simulink model "pure_inematic"  (R2020b)
settings: Solver=FixedStepAuto  StartTime=0.0  StopTime=40  FixedStep=0.001  RelTol=1e-3
settings Model: Creator=cyx  LastModifiedBy=cyx
settings DataIOCC: ReturnWorkspaceOutputs=off

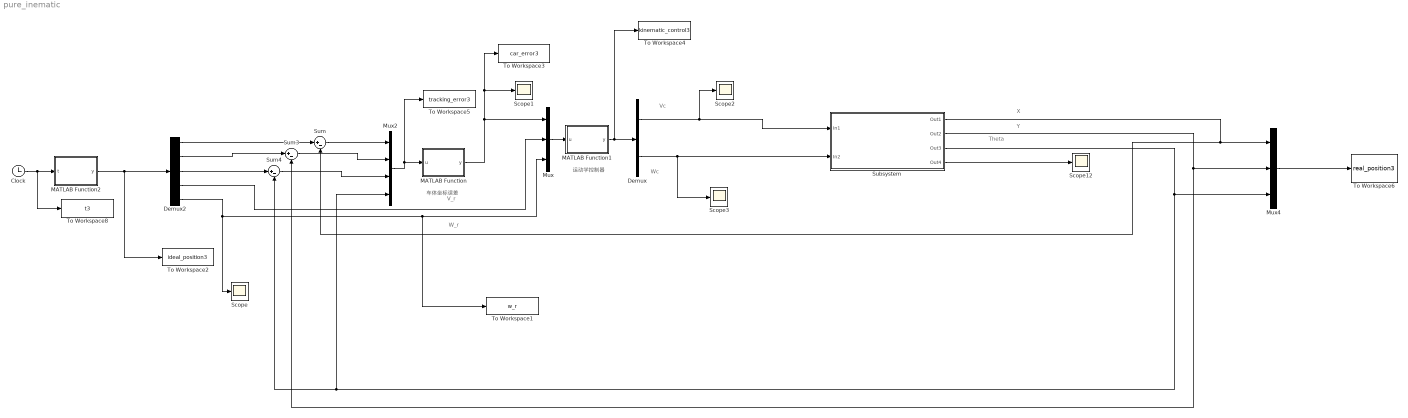
== system pure_inematic ==
  note: 运动学控制器
  note: Theta
  note: Wc
  note: X
  note: V_r
  note: Vc
  note: W_r
  note: 车体坐标误差
  note: Y
  Clock : Clock
  Demux : Demux  Outputs=[1 1]
  Demux2 : Demux  Outputs=5
  MATLAB Function : MATLAB Function  TreatAsAtomicUnit=on
  MATLAB Function1 : MATLAB Function  TreatAsAtomicUnit=on
  MATLAB Function2 : MATLAB Function  TreatAsAtomicUnit=on
  Mux : Mux  Inputs=3
  Mux2 : Mux  Inputs=[1 1 1 1]
  Mux4 : Mux  Inputs=3
  Scope{,1..3,12} (5 alike) : Scope
  Subsystem : Subsystem
  Sum : Sum  Inputs=|+-
  Sum3 : Sum  Inputs=|+-
  Sum4 : Sum  Inputs=|+-
  To Workspace1 : ToWorkspace  VariableName=w_r  SampleTime=-1
  To Workspace2 : ToWorkspace  VariableName=ideal_position3  SampleTime=-1
  To Workspace3 : ToWorkspace  VariableName=car_error3  SampleTime=-1
  To Workspace4 : ToWorkspace  VariableName=kinematic_control3  SampleTime=-1
  To Workspace5 : ToWorkspace  VariableName=tracking_error3  SampleTime=-1
  To Workspace6 : ToWorkspace  VariableName=real_position3  SampleTime=-1
      settings: Save2DSignal=2-D array (concatenate along first dimension)
  To Workspace8 : ToWorkspace  VariableName=t3  SampleTime=-1
  wires:
  Mux4/1 -> To Workspace6/1
  Demux2/3 -> Sum4/1
  Subsystem/1(Out1) -> Mux4/1, Sum/2
  MATLAB Function2/1(y) -> To Workspace2/1, Demux2/1
  Demux2/4 -> Mux/2
  Clock/1 -> To Workspace8/1, MATLAB Function2/1(t)
  Subsystem/3(Out3) -> Mux4/3, Mux2/4, Sum4/2
  Sum/1 -> Mux2/1
  Subsystem/4(Out4) -> Scope12/1
  Sum3/1 -> Mux2/2
  Mux2/1 -> To Workspace5/1, MATLAB Function/1(u)
  Sum4/1 -> Mux2/3
  Demux2/1 -> Sum/1
  Mux/1 -> MATLAB Function1/1(u)
  Demux2/2 -> Sum3/1
  Subsystem/2(Out2) -> Mux4/2, Sum3/2
  MATLAB Function/1(y) -> To Workspace3/1, Scope1/1, Mux/1
  MATLAB Function1/1(y) -> To Workspace4/1, Demux/1
  Demux/1 -> Scope2/1, Subsystem/1(In1)
  Demux/2 -> Scope3/1, Subsystem/2(In2)
  Demux2/5 -> To Workspace1/1, Mux/3, Scope/1

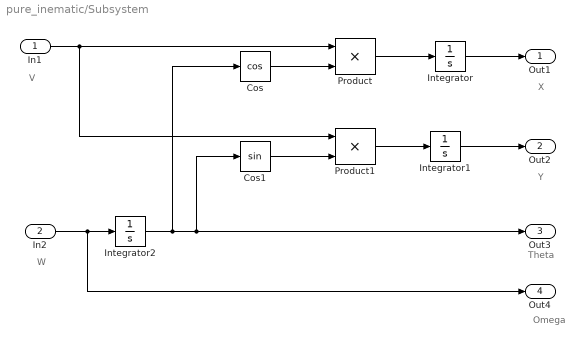
== system pure_inematic/Subsystem ==
  note: W
  note: V
  note: X
  note: Y
  note: Theta
  note: Omega
  In1 : Inport
  In2 : Inport  Port=2
  Cos : Trigonometry  Operator=cos
  Cos1 : Trigonometry
  Integrator : Integrator  InitialCondition=-2
  Integrator1 : Integrator  InitialCondition=-2
  Integrator2 : Integrator
  Product : Product
  Product1 : Product
  Out1 : Outport
  Out2 : Outport  Port=2
  Out3 : Outport  Port=3
  Out4 : Outport  Port=4
  wires:
  In1/1 -> Product1/1, Product/1
  Product/1 -> Integrator/1
  Integrator/1 -> Out1/1
  Cos/1 -> Product/2
  Integrator1/1 -> Out2/1
  In2/1 -> Out4/1, Integrator2/1
  Integrator2/1 -> Cos1/1, Out3/1, Cos/1
  Product1/1 -> Integrator1/1
  Cos1/1 -> Product1/2

== matlab function pure_inematic/MATLAB Function ==
  data: u input; y output
function y = error(u)
%%讲机器人误差坐标进行转换；
%转换矩阵C

C=[cos(u(4))   sin(u(4))    0;
   -sin(u(4)) cos(u(4))    0;
    0            0          1];

%%将世界坐标系下的误差转化至车体坐标下转换后的误差q_e=[e1 e2 e3]
%输入为世界坐标系下的误差x_e,y_e,theta_e对应u(1),u(2) u(3)
e1=C(1,1)*u(1)+C(1,2)*u(2);
e2=C(2,1)*u(1)+C(2,2)*u(2);
e3=C(3,3)*u(3);
y =[e1;e2;e3];

== matlab function pure_inematic/MATLAB Function2 ==
  data: t input; y output
function y = input(t)

S=3;
switch S

   case 1 %圆形轨迹
       w_r=1;
       x_r= 5*cos(w_r*t);
       y_r= 5+5*sin(w_r*t);
       theta_r=w_r*t;
        v_r=5;
               
    case 2 %8轨迹
        x_r=10*sin(t/10);
        y_r=10*sin(t/20);
        dx_r=cos(t/10);
        dy_r=0.5*cos(t/20);
        if atan2(dy_r,dx_r)>0
            theta_r=atan2(dy_r,dx_r);
        else
            theta_r=atan2(dy_r,dx_r)+2*pi;
        end
        v_r=sqrt(dy_r.^2+dx_r.^2);
        w_r=0.5;

    case 3 %rectangle
        x_r=sign(cos(t)).*sqrt(abs(100*cos(t)));
        y_r=sign(sin(t)).*sqrt(abs(100*sin(t)));
        theta_r=atan2(y_r,x_r);
        if 0<t && t<3.146 | 10<t && t<13.146 | 20<t && t<23.146 | 30<t && t<33.146
            v_r=0.8;
            w_r=0.5;
        else
            v_r=1;
            w_r=0;
        end
 
end


y =[x_r; y_r; theta_r; v_r; w_r];

== matlab function pure_inematic/MATLAB Function1 ==
  data: u input; y output
function y = kinematic(u)
ex=u(1);
ey=u(2);
etheta=u(3);
v_r=u(4);
w_r=u(5);
%%机器人反演控制律；控制输入为参考速度v_r,w_r以及三个车体坐标系误差；
%k1=123; k2=1;k3=23;
%v_c=v_r*cos(etheta)+k1*ex;
%w_c=w_r+k2*v_r*ey+k3*v_r*sin(etheta);

%k1=0.01;k2=16;k3=4;k4=16;vr_dot=0;wr_dot=0;
%w_c=k2*ey*v_r*cos(etheta/2)*cos(etheta/4)+w_r+k4*sin(etheta/4);
%v_c=v_r*cos(etheta)-k1*ey/(1+w_c.^2)*(k2*((-w_c*ex+v_r*sin(etheta)*v_r+ey*vr_dot)*cos(etheta/2)*cos(etheta/4)-...
 %  (k2*ey*v_r*sin(etheta/4)*(0.5+0.75*cos(etheta/2)-0.25*k4*cos(etheta)*(w_r-w_c))...
 %   +wr_dot-k1*atan(w_c)*(-w_c*ex+v_r*sin(etheta))+...
  %  k3*abs(ex-k1*atan(w_c)*ey)*sign(ex-k1*atan(w_c)*ey))));
    
%反步法设计控制律2
%k1=0.5;k2=300;k3=400;k4=10;
%w_c=k2*ey*v_r*cos(etheta/2)*cos(etheta/4)+k4*sin(etheta/4)+w_r;
%e1_bar=ex-k1*atan(w_r)*ey;
%vrdot=0;
%wrdot=0;
%w_cdot=k2*((-w_r*ex+v_r*sin(etheta))*v_r+ey*vrdot)*cos(etheta/2)...
  %   *cos(etheta/4)-(k2*ey*v_r*sin(etheta/4)*(0.5+0.75*cos(etheta/2))-0.25*k4*cos(etheta/4))...
  %   *(w_r-w_r)+wrdot;
%v_c=v_r*cos(etheta)-k1*ey/(1+w_r^2)*w_cdot-k1*atan(w_r)*(-w_r*ex+v_r*sin(etheta))+k3*e1_bar;


%k1=6;k2=2;k3=2;
%v_c=v_r+k2*power(abs(ex),2/3)*sign(ex)-k3*w_r*power(abs(ey),1/3)*sign(ey);
%w_c=w_r+k1*power(abs(etheta),1/3)*sign(etheta);




%反步法设计控制律3
k1=0.1;k2=100;k3=150;k4=10;
w_c=2*k3*ey*v_r*cos(etheta/2)+k4*sin(etheta/2)+w_r;
%e1_bar=e1-k1*(omega/(1+omega^2)^0.5)*e2;
vrdot=0;
wrdot=0;
omega_dot=2*k3*((-w_c*ex+v_r*sin(etheta))*v_r+ey*vrdot)*cos(etheta/2)-k3*ey*v_r*sin(etheta/2)*(w_r-w_c)...
    +0.5*k4*cos(etheta/2)*(w_r-w_c)+wrdot;
v_c=v_r*cos(etheta)+k1*w_c*ex*(w_c/(1+w_c^2)^0.5)-k1*v_r*sin(etheta)*(w_c/(1+w_c^2)^0.5)...
    -k1*omega_dot*ey/(1+w_c^2)^1.5+k2*(ex-k1*ey*(w_c/(1+w_c^2)^0.5));


%if abs(v_c)>10
  %  v_c=sign(v_c)*10;
%end
%if abs(w_c)>10
%    w_c=sign(w_c)*10;
%end

%gama=10;k=20;
%phi1=power(ex,3)+k*ex+nthroot(ex,3); 
%phi2=power(ey,3)+k*ey+nthroot(ey,3);
%phi3=power(etheta,3)+k*etheta+nthroot(etheta,3);

%控制率u-------------------------------------------------------------------
%v_c=ey*((w_r+gama*phi3+v_r*sin(etheta)+gama*phi2)/(ex+1))+v_r*cos(etheta)+gama*phi1;
%w_c=((w_r+gama*phi3+v_r*sin(etheta)+gama*phi2)/(ex+1));%w

if abs(v_c)>10
    v_c=sign(v_c)*10;
end
if abs(w_c)>10
    w_c=sign(w_c)*10;
end


y = [v_c;w_c];
